simulink model "FSK_1"  (R2017b)
settings: Solver=VariableStepAuto  StartTime=0.0  StopTime=10.0  MaxStep=0.01  MinStep=0.001  RelTol=1e-3
libraries: dsparch4 x2
settings Model: Creator=ayadd  LastModifiedBy=ayadd
settings SolverCC: ShapePreserveControl=EnableAll  ZeroCrossAlgorithm=Adaptive

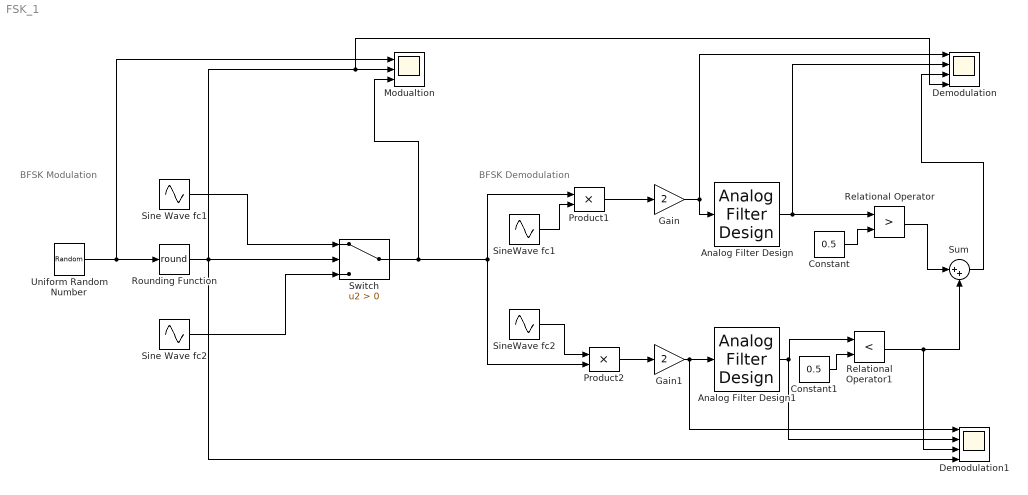
== system FSK_1 ==
  note: BFSK Demodulation
  note: BFSK Modulation
  Analog Filter Design : dsparch4/Analog Filter Design  method=Butterworth  filttype=Lowpass  N=8  Wlo=30  Whi=80  Rp=2  Rs=40
  Analog Filter Design1 : dsparch4/Analog Filter Design  method=Butterworth  filttype=Lowpass  N=8  Wlo=30  Whi=80  Rp=2  Rs=40
  Constant : Constant  Value=0.5
  Constant1 : Constant  Value=0.5
  Demodulation : Scope  NumInputPorts=4
  Demodulation1 : Scope  NumInputPorts=4
  Gain : Gain  Gain=2
  Gain1 : Gain  Gain=2
  Modualtion : Scope  NumInputPorts=3
  Product1 : Product  SaturateOnIntegerOverflow=on  InputSameDT=on  OutDataTypeStr=Inherit: Same as first input
  Product2 : Product  SaturateOnIntegerOverflow=on  InputSameDT=on  OutDataTypeStr=Inherit: Same as first input
  Relational Operator : RelationalOperator  Operator=>  RndMeth=Nearest  InputSameDT=on
  Relational Operator1 : RelationalOperator  Operator=<  RndMeth=Nearest  InputSameDT=on
  Rounding Function : Rounding  Operator=round
  Sine Wave fc1 : Sin  Frequency=15*2*pi  SampleTime=0
  Sine Wave fc2 : Sin  Frequency=5*2*pi  SampleTime=0
  SineWave fc1 : Sin  Frequency=15*2*pi  SampleTime=0
  SineWave fc2 : Sin  Frequency=5*2*pi  SampleTime=0
  Sum : Sum  Inputs=|++
  Switch : Switch  Criteria=u2 > Threshold
  Uniform Random Number : UniformRandomNumber  Minimum=0  SampleTime=1
  wires:
  Uniform Random Number/1 -> Modualtion/1, Rounding Function/1
  Sine Wave fc2/1 -> Switch/3
  SineWave fc1/1 -> Product1/2
  Product1/1 -> Gain/1
  Analog Filter Design/1 -> Demodulation/2, Relational Operator/1
  Constant/1 -> Relational Operator/2
  Gain/1 -> Analog Filter Design/1, Demodulation/1
  Rounding Function/1 -> Demodulation1/4, Switch/2, Demodulation/4, Modualtion/2
  Sine Wave fc1/1 -> Switch/1
  SineWave fc2/1 -> Product2/1
  Constant1/1 -> Relational Operator1/2
  Gain1/1 -> Demodulation1/1, Analog Filter Design1/1
  Analog Filter Design1/1 -> Demodulation1/2, Relational Operator1/1
  Product2/1 -> Gain1/1
  Relational Operator/1 -> Sum/1
  Relational Operator1/1 -> Demodulation1/3, Sum/2
  Switch/1 -> Modualtion/3, Product2/2, Product1/1
  Sum/1 -> Demodulation/3
